simulink model "loop"  (R2024b)
settings: Solver=VariableStepAuto  StartTime=0.0  StopTime=10.0  RelTol=1e-3
settings Model: Creator=ryandavis  LastModifiedBy=ryandavis

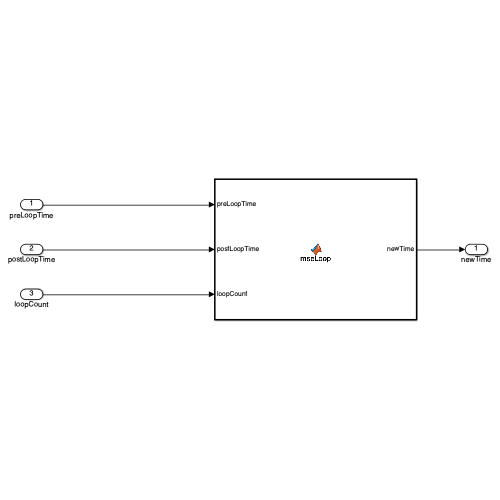
[thumbnail: Simulink's stored preview of the top-level diagram]
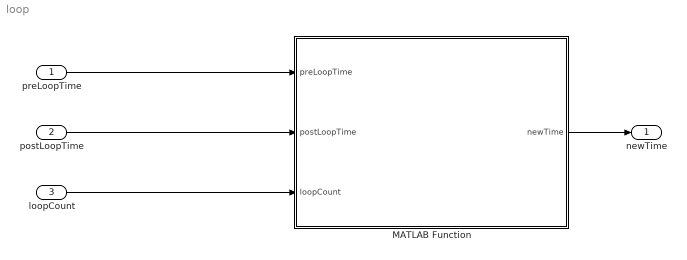
== system loop ==
  preLoopTime : Inport
  postLoopTime : Inport  Port=2
  loopCount : Inport  Port=3
  MATLAB Function : MATLAB Function  TreatAsAtomicUnit=on
  newTime : Outport
  wires:
  postLoopTime/1 -> MATLAB Function/2(postLoopTime)
  loopCount/1 -> MATLAB Function/3(loopCount)
  preLoopTime/1 -> MATLAB Function/1(preLoopTime)
  MATLAB Function/1(newTime) -> newTime/1

== matlab function loop/MATLAB Function ==
  data: preLoopTime input; newTime output; postLoopTime input; loopCount input
function newTime= mseLoop(preLoopTime, postLoopTime, loopCount)
newTime= preLoopTime+loopCount*(postLoopTime-preLoopTime);
